simulink model "fiveSec"  (R2019b)
settings: Solver=ode5  StartTime=0.0  StopTime=56  FixedStep=1/1000  RelTol=1e-3
libraries: simulink x1
settings Model: Creator=Çevikalp Sütunç  LastModifiedBy=Çevikalp Sütunç

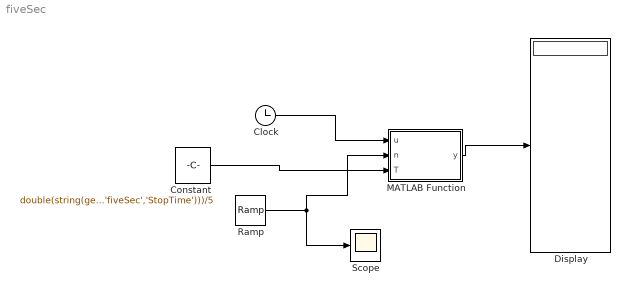
== system fiveSec ==
  Clock : Clock
  Constant : Constant  Value=double(string(get_param('fiveSec','StopTime')))/5
  Display : Display
  MATLAB Function : MATLAB Function  TreatAsAtomicUnit=on
  Ramp : simulink/Sources/Ramp  slope=0.26  start=0  InitialOutput=0
  Scope : Scope
  wires:
  Clock/1 -> MATLAB Function/1(u)
  Ramp/1 -> MATLAB Function/2(n), Scope/1
  MATLAB Function/1(y) -> Display/1
  Constant/1 -> MATLAB Function/3(T)

== matlab function fiveSec/MATLAB Function ==
  settings: updateMethod=DISCRETE  sampleTime=0.001
  data: u input; y output size=[1 floor(double(string(get_param('fiveSec','StopTime')))/5)+1]; n input; T input
function y  = fcn(u,n,T)
y=zeros(1,floor(T)+1);
i=0;
persistent I Y
if isempty(I)
    I=double(0);
end
if isempty(Y)
    Y=zeros(1,floor(T)+1);
end
if mod(u,5)==0
    I=I+1;
    i=I;
    Y(i)=n;
    y(i)=Y(i);
end
y=Y;
i=I;
end
